simulink model "Task_Space_Trajectory"  (R2019b)
settings: Solver=FixedStepAuto  StartTime=0.0  StopTime=8  FixedStep=0.01  RelTol=1e-3
libraries: simulink x1
settings Model: Creator=gasserelazab  LastModifiedBy=gasserelazab

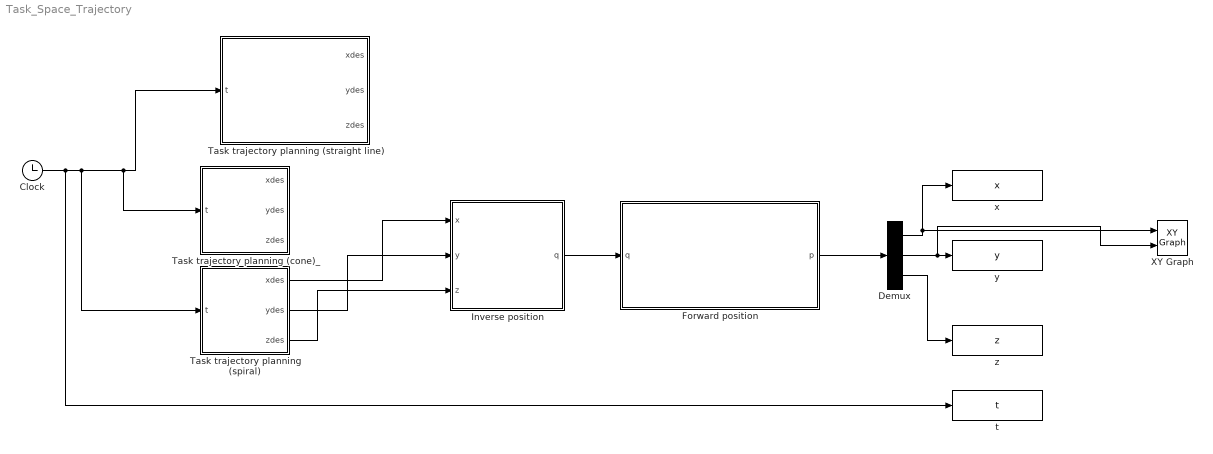
== system Task_Space_Trajectory ==
  Clock : Clock
  Demux : Demux  Outputs=3
  "Forward position " : MATLAB Function  TreatAsAtomicUnit=on
  "Inverse position " : MATLAB Function  TreatAsAtomicUnit=on
  "Task trajectory planning (cone)_ " : MATLAB Function  TreatAsAtomicUnit=on
  "Task trajectory planning (spiral) " : MATLAB Function  TreatAsAtomicUnit=on
  "Task trajectory planning (straight line) " : MATLAB Function  TreatAsAtomicUnit=on
  XY Graph : simulink/Sinks/XY Graph  xmin=-50  xmax=50  ymin=-50  ymax=50  st=-1
  t : ToWorkspace  VariableName=t  SampleTime=0.01
  "x " : ToWorkspace  VariableName=x  SampleTime=0.01
  y : ToWorkspace  VariableName=y  SampleTime=0.01
  z : ToWorkspace  VariableName=z  SampleTime=0.01
  wires:
  Clock/1 -> t/1, "Task trajectory planning (spiral) "/1(t), "Task trajectory planning (cone)_ "/1(t), "Task trajectory planning (straight line) "/1(t)
  "Inverse position "/1(q) -> "Forward position "/1(q)
  "Forward position "/1(p) -> Demux/1
  Demux/1 -> "x "/1, XY Graph/1
  Demux/2 -> XY Graph/2, y/1
  Demux/3 -> z/1
  "Task trajectory planning (spiral) "/1(xdes) -> "Inverse position "/1(x)
  "Task trajectory planning (spiral) "/2(ydes) -> "Inverse position "/2(y)
  "Task trajectory planning (spiral) "/3(zdes) -> "Inverse position "/3(z)

== matlab function Task_Space_Trajectory/Inverse position  ==
  data: q output; x input; y input; z input
function q   = fcn(x, y, z)

qnew=[0;0;0;0;0;0];
qold=[50;50;50;50;50;50];

i=100;
dog=true;

while (i>0 && dog)
    q1=qold(1,1);
    q2=qold(2,1);
    q3=qold(3,1);
    q4=qold(4,1);
    q5=qold(5,1);
    q6=qold(6,1);
    
    F= [ 10*cos((pi*(q1 - 90))/180)*sin((pi*(q2 - 90))/180) - 10*sin((pi*(q5 + 90))/180)*(sin((pi*(q1 - 90))/180)*sin((pi*(q4 + 90))/180) - cos((pi*(q1 - 90))/180)*cos((pi*(q2 - 90))/180)*cos((pi*(q4 + 90))/180)) - x + cos((pi*(q1 - 90))/180)*sin((pi*(q2 - 90))/180)*(q3 + 10) - 10*cos((pi*(q1 - 90))/180)*cos((pi*(q5 + 90))/180)*sin((pi*(q2 - 90))/180);...
 10*sin((pi*(q5 + 90))/180)*(cos((pi*(q1 - 90))/180)*sin((pi*(q4 + 90))/180) + cos((pi*(q2 - 90))/180)*cos((pi*(q4 + 90))/180)*sin((pi*(q1 - 90))/180)) - y + 10*sin((pi*(q1 - 90))/180)*sin((pi*(q2 - 90))/180) + sin((pi*(q1 - 90))/180)*sin((pi*(q2 - 90))/180)*(q3 + 10) - 10*cos((pi*(q5 + 90))/180)*sin((pi*(q1 - 90))/180)*sin((pi*(q2 - 90))/180);...
                                                                                                                                                10*cos((pi*(q2 - 90))/180) - z + cos((pi*(q2 - 90))/180)*(q3 + 10) - 10*cos((pi*(q2 - 90))/180)*cos((pi*(q5 + 90))/180) - 10*cos((pi*(q4 + 90))/180)*sin((pi*(q2 - 90))/180)*sin((pi*(q5 + 90))/180) + 10];
 FJ= [ (pi*cos((pi*(q5 + 90))/180)*sin((pi*(q1 - 90))/180)*sin((pi*(q2 - 90))/180))/18 - (pi*sin((pi*(q1 - 90))/180)*sin((pi*(q2 - 90))/180))/18 - (pi*sin((pi*(q1 - 90))/180)*sin((pi*(q2 - 90))/180)*(q3 + 10))/180 - 10*sin((pi*(q5 + 90))/180)*((pi*cos((pi*(q1 - 90))/180)*sin((pi*(q4 + 90))/180))/180 + (pi*cos((pi*(q2 - 90))/180)*cos((pi*(q4 + 90))/180)*sin((pi*(q1 - 90))/180))/180), (pi*cos((pi*(q1 - 90))/180)*cos((pi*(q2 - 90))/180))/18 + (pi*cos((pi*(q1 - 90))/180)*cos((pi*(q2 - 90))/180)*(q3 + 10))/180 - (pi*cos((pi*(q1 - 90))/180)*cos((pi*(q2 - 90))/180)*cos((pi*(q5 + 90))/180))/18 - (pi*cos((pi*(q1 - 90))/180)*cos((pi*(q4 + 90))/180)*sin((pi*(q2 - 90))/180)*sin((pi*(q5 + 90))/180))/18, cos((pi*(q1 - 90))/180)*sin((pi*(q2 - 90))/180), -10*sin((pi*(q5 + 90))/180)*((pi*cos((pi*(q4 + 90))/180)*sin((pi*(q1 - 90))/180))/180 + (pi*cos((pi*(q1 - 90))/180)*cos((pi*(q2 - 90))/180)*sin((pi*(q4 + 90))/180))/180), (pi*cos((pi*(q1 - 90))/180)*sin((pi*(q2 - 90))/180)*sin((pi*(q5 + 90))/180))/18 - (pi*cos((pi*(q5 + 90))/180)*(sin((pi*(q1 - 90))/180)*sin((pi*(q4 + 90))/180) - cos((pi*(q1 - 90))/180)*cos((pi*(q2 - 90))/180)*cos((pi*(q4 + 90))/180)))/18, 0;...
 (pi*cos((pi*(q1 - 90))/180)*sin((pi*(q2 - 90))/180))/18 - 10*sin((pi*(q5 + 90))/180)*((pi*sin((pi*(q1 - 90))/180)*sin((pi*(q4 + 90))/180))/180 - (pi*cos((pi*(q1 - 90))/180)*cos((pi*(q2 - 90))/180)*cos((pi*(q4 + 90))/180))/180) + (pi*cos((pi*(q1 - 90))/180)*sin((pi*(q2 - 90))/180)*(q3 + 10))/180 - (pi*cos((pi*(q1 - 90))/180)*cos((pi*(q5 + 90))/180)*sin((pi*(q2 - 90))/180))/18, (pi*cos((pi*(q2 - 90))/180)*sin((pi*(q1 - 90))/180))/18 + (pi*cos((pi*(q2 - 90))/180)*sin((pi*(q1 - 90))/180)*(q3 + 10))/180 - (pi*cos((pi*(q2 - 90))/180)*cos((pi*(q5 + 90))/180)*sin((pi*(q1 - 90))/180))/18 - (pi*cos((pi*(q4 + 90))/180)*sin((pi*(q1 - 90))/180)*sin((pi*(q2 - 90))/180)*sin((pi*(q5 + 90))/180))/18, sin((pi*(q1 - 90))/180)*sin((pi*(q2 - 90))/180),  10*sin((pi*(q5 + 90))/180)*((pi*cos((pi*(q1 - 90))/180)*cos((pi*(q4 + 90))/180))/180 - (pi*cos((pi*(q2 - 90))/180)*sin((pi*(q1 - 90))/180)*sin((pi*(q4 + 90))/180))/180), (pi*cos((pi*(q5 + 90))/180)*(cos((pi*(q1 - 90))/180)*sin((pi*(q4 + 90))/180) + cos((pi*(q2 - 90))/180)*cos((pi*(q4 + 90))/180)*sin((pi*(q1 - 90))/180)))/18 + (pi*sin((pi*(q1 - 90))/180)*sin((pi*(q2 - 90))/180)*sin((pi*(q5 + 90))/180))/18, 0;...
                                                                                                                                                                                                                                                                                                                                                                                         0,                                                                                                 (pi*cos((pi*(q5 + 90))/180)*sin((pi*(q2 - 90))/180))/18 - (pi*sin((pi*(q2 - 90))/180)*(q3 + 10))/180 - (pi*sin((pi*(q2 - 90))/180))/18 - (pi*cos((pi*(q2 - 90))/180)*cos((pi*(q4 + 90))/180)*sin((pi*(q5 + 90))/180))/18,                         cos((pi*(q2 - 90))/180),                                                                                           (pi*sin((pi*(q2 - 90))/180)*sin((pi*(q4 + 90))/180)*sin((pi*(q5 + 90))/180))/18,                                                                                                     (pi*cos((pi*(q2 - 90))/180)*sin((pi*(q5 + 90))/180))/18 - (pi*cos((pi*(q4 + 90))/180)*cos((pi*(q5 + 90))/180)*sin((pi*(q2 - 90))/180))/18, 0];
 

    inverseFJ= transpose(FJ)*(inv(FJ*transpose(FJ)));
        
 
    qnew=qold-inverseFJ*F;
    %disp(inverseFJ*F);
    
  
   
    count=0;
   
   	for xx = 1:6
        if  ((qnew(xx,1)-qold(xx,1)<0.1) && (qnew(xx,1)-qold(xx,1)>-0.1 ))       
             count=count+1;
         end
   
    end
    
    if( count == 6)
        dog=false;
    end
    
    i=i-1;
    
    %disp(i);
    
    qold=qnew;
    
end
q=qold;

== matlab function Task_Space_Trajectory/Task trajectory planning (straight line)  ==
  data: t input; xdes output; ydes output; zdes output
function [xdes, ydes, zdes] = fcn(t)

xdes= 3-0.5*t;
ydes= 5-0.375*t;
zdes= 7-0.375*t;

== matlab function Task_Space_Trajectory/Forward position  ==
  data: p output; q input
function p  = fcn(q)
q1= q(1);
q2= q(2);
q3= q(3);
q4= q(4);
q5= q(5);
q6= q(6);
L1=10;
L2=10;
L3=10;
L4=10;
pp= [ sin((pi*q6)/180)*(cos((pi*(q4 + 90))/180)*sin((pi*(q1 - 90))/180) + cos((pi*(q1 - 90))/180)*cos((pi*(q2 - 90))/180)*sin((pi*(q4 + 90))/180)) - cos((pi*q6)/180)*(cos((pi*(q5 + 90))/180)*(sin((pi*(q1 - 90))/180)*sin((pi*(q4 + 90))/180) - cos((pi*(q1 - 90))/180)*cos((pi*(q2 - 90))/180)*cos((pi*(q4 + 90))/180)) - cos((pi*(q1 - 90))/180)*sin((pi*(q2 - 90))/180)*sin((pi*(q5 + 90))/180)),   sin((pi*q6)/180)*(cos((pi*(q5 + 90))/180)*(sin((pi*(q1 - 90))/180)*sin((pi*(q4 + 90))/180) - cos((pi*(q1 - 90))/180)*cos((pi*(q2 - 90))/180)*cos((pi*(q4 + 90))/180)) - cos((pi*(q1 - 90))/180)*sin((pi*(q2 - 90))/180)*sin((pi*(q5 + 90))/180)) + cos((pi*q6)/180)*(cos((pi*(q4 + 90))/180)*sin((pi*(q1 - 90))/180) + cos((pi*(q1 - 90))/180)*cos((pi*(q2 - 90))/180)*sin((pi*(q4 + 90))/180)), - sin((pi*(q5 + 90))/180)*(sin((pi*(q1 - 90))/180)*sin((pi*(q4 + 90))/180) - cos((pi*(q1 - 90))/180)*cos((pi*(q2 - 90))/180)*cos((pi*(q4 + 90))/180)) - cos((pi*(q1 - 90))/180)*cos((pi*(q5 + 90))/180)*sin((pi*(q2 - 90))/180), cos((pi*(q1 - 90))/180)*sin((pi*(q2 - 90))/180)*(L2 + q3) - L4*(sin((pi*(q5 + 90))/180)*(sin((pi*(q1 - 90))/180)*sin((pi*(q4 + 90))/180) - cos((pi*(q1 - 90))/180)*cos((pi*(q2 - 90))/180)*cos((pi*(q4 + 90))/180)) + cos((pi*(q1 - 90))/180)*cos((pi*(q5 + 90))/180)*sin((pi*(q2 - 90))/180)) + L3*cos((pi*(q1 - 90))/180)*sin((pi*(q2 - 90))/180);
 cos((pi*q6)/180)*(cos((pi*(q5 + 90))/180)*(cos((pi*(q1 - 90))/180)*sin((pi*(q4 + 90))/180) + cos((pi*(q2 - 90))/180)*cos((pi*(q4 + 90))/180)*sin((pi*(q1 - 90))/180)) + sin((pi*(q1 - 90))/180)*sin((pi*(q2 - 90))/180)*sin((pi*(q5 + 90))/180)) - sin((pi*q6)/180)*(cos((pi*(q1 - 90))/180)*cos((pi*(q4 + 90))/180) - cos((pi*(q2 - 90))/180)*sin((pi*(q1 - 90))/180)*sin((pi*(q4 + 90))/180)), - sin((pi*q6)/180)*(cos((pi*(q5 + 90))/180)*(cos((pi*(q1 - 90))/180)*sin((pi*(q4 + 90))/180) + cos((pi*(q2 - 90))/180)*cos((pi*(q4 + 90))/180)*sin((pi*(q1 - 90))/180)) + sin((pi*(q1 - 90))/180)*sin((pi*(q2 - 90))/180)*sin((pi*(q5 + 90))/180)) - cos((pi*q6)/180)*(cos((pi*(q1 - 90))/180)*cos((pi*(q4 + 90))/180) - cos((pi*(q2 - 90))/180)*sin((pi*(q1 - 90))/180)*sin((pi*(q4 + 90))/180)),   sin((pi*(q5 + 90))/180)*(cos((pi*(q1 - 90))/180)*sin((pi*(q4 + 90))/180) + cos((pi*(q2 - 90))/180)*cos((pi*(q4 + 90))/180)*sin((pi*(q1 - 90))/180)) - cos((pi*(q5 + 90))/180)*sin((pi*(q1 - 90))/180)*sin((pi*(q2 - 90))/180), L4*(sin((pi*(q5 + 90))/180)*(cos((pi*(q1 - 90))/180)*sin((pi*(q4 + 90))/180) + cos((pi*(q2 - 90))/180)*cos((pi*(q4 + 90))/180)*sin((pi*(q1 - 90))/180)) - cos((pi*(q5 + 90))/180)*sin((pi*(q1 - 90))/180)*sin((pi*(q2 - 90))/180)) + sin((pi*(q1 - 90))/180)*sin((pi*(q2 - 90))/180)*(L2 + q3) + L3*sin((pi*(q1 - 90))/180)*sin((pi*(q2 - 90))/180);
                                                                                                                                                                                 cos((pi*q6)/180)*(cos((pi*(q2 - 90))/180)*sin((pi*(q5 + 90))/180) - cos((pi*(q4 + 90))/180)*cos((pi*(q5 + 90))/180)*sin((pi*(q2 - 90))/180)) - sin((pi*q6)/180)*sin((pi*(q2 - 90))/180)*sin((pi*(q4 + 90))/180),                                                                                                                                                                                 - sin((pi*q6)/180)*(cos((pi*(q2 - 90))/180)*sin((pi*(q5 + 90))/180) - cos((pi*(q4 + 90))/180)*cos((pi*(q5 + 90))/180)*sin((pi*(q2 - 90))/180)) - cos((pi*q6)/180)*sin((pi*(q2 - 90))/180)*sin((pi*(q4 + 90))/180),                                                                                                     - cos((pi*(q2 - 90))/180)*cos((pi*(q5 + 90))/180) - cos((pi*(q4 + 90))/180)*sin((pi*(q2 - 90))/180)*sin((pi*(q5 + 90))/180),                                                                                                                                                L1 - L4*(cos((pi*(q2 - 90))/180)*cos((pi*(q5 + 90))/180) + cos((pi*(q4 + 90))/180)*sin((pi*(q2 - 90))/180)*sin((pi*(q5 + 90))/180)) + cos((pi*(q2 - 90))/180)*(L2 + q3) + L3*cos((pi*(q2 - 90))/180);
                                                                                                                                                                                                                                                                                                                                                                                               0,                                                                                                                                                                                                                                                                                                                                                                                                 0,                                                                                                                                                                                                                               0,                                                                                                                                                                                                                                                                                                                                                   1];
x=pp(1,4);
y=pp(2,4);
z=pp(3,4);
p= [x;y;z];

== matlab function Task_Space_Trajectory/Task trajectory planning (cone)_  ==
  data: t input; xdes output; ydes output; zdes output
function [xdes,ydes,zdes]= fcn(t)
xdes=(20-2.375*t)*cos(pi*t);
ydes=(20-2.375*t)*sin(pi*t);
zdes=10+3.75*t;

== matlab function Task_Space_Trajectory/Task trajectory planning (spiral)  ==
  data: t input; xdes output; ydes output; zdes output
function [xdes,ydes,zdes]= fcn(t)
xdes=(20-0.25*t)*cos(pi*t);
ydes=(5-0.25*t)*sin(pi*t);
zdes=10+0.5*t;
